simulink model "seven_level_NPC_MLI_Inverter"  (R2022a)
settings: Solver=VariableStepAuto  StartTime=0.0  StopTime=0.02  RelTol=1e-3
libraries: spsDiodeLib x30, spsVoltageMeasurementLib x13, spsIGBTDiodeLib x12, spsDCVoltageSourceLib x6, simulink x6, spsCurrentMeasurementLib x1, spsSeriesRLCBranchLib x1, spspowerguiLib x1
settings Model: Creator=P.O.M.G  LastModifiedBy=P.O.M.G

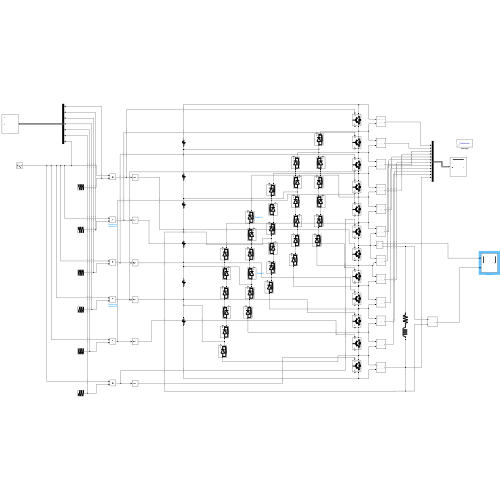
[thumbnail: Simulink's stored preview of the top-level diagram]
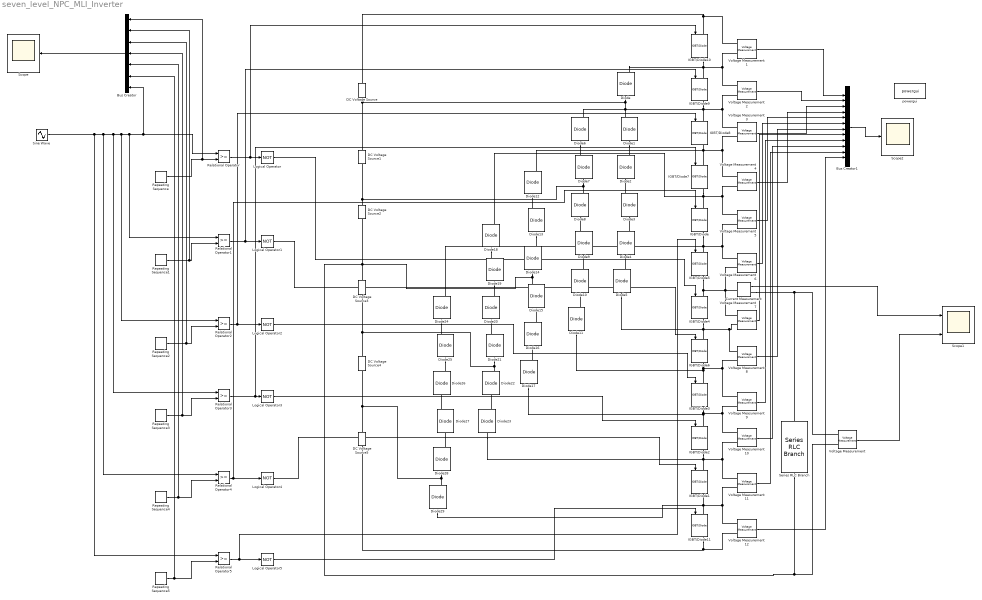
== system seven_level_NPC_MLI_Inverter ==
  Bus Creator : BusCreator  Inputs=7
  Bus Creator1 : BusCreator  Inputs=12
  Current Measurement : spsCurrentMeasurementLib/Current Measurement  PhasorSimulation=off  OutputType=Complex  PSBequivalent=0
  DC Voltage Source{,1..5} (6 alike) : spsDCVoltageSourceLib/DC Voltage Source  Amplitude=100  Measurements=None
  Diode{,1..29} (30 alike) : spsDiodeLib/Diode  Ron=0.001  Lon=0  Vf=0.8  IC=0  UseSnubber=0  Rs=500  Cs=250e-9  Measurements=on
  IGBT/Diode{,1..11} (12 alike) : spsIGBTDiodeLib/IGBT//Diode  Ron=1e-3  Rs=1e5  Cs=inf  Measurements=on
  Logical Operator{,1..5} (6 alike) : Logic  Operator=NOT  AllPortsSameDT=off  OutDataTypeStr=boolean
  Relational Operator{,1..5} (6 alike) : RelationalOperator  OutDataTypeStr=boolean  RndMeth=Simplest  InputSameDT=off
  Repeating Sequence : simulink/Sources/Repeating Sequence  rep_seq_t=[0 0.5 1]/500  rep_seq_y=[1, 0, -1]
  Repeating Sequence1 : simulink/Sources/Repeating Sequence  rep_seq_t=[0 0.5 1]/500  rep_seq_y=[0, 1, -1]
  Repeating Sequence2 : simulink/Sources/Repeating Sequence  rep_seq_t=[0 0.5 1]/500  rep_seq_y=[-1, 1, 0]
  Repeating Sequence3 : simulink/Sources/Repeating Sequence  rep_seq_t=[0 0.5 1]/500  rep_seq_y=[-1, 0, 1]
  Repeating Sequence4 : simulink/Sources/Repeating Sequence  rep_seq_t=[0 0.5 1]/500  rep_seq_y=[1, -1, 0]
  Repeating Sequence5 : simulink/Sources/Repeating Sequence  rep_seq_t=[0 0.5 1]/500  rep_seq_y=[0, -1, 1]
  Scope : Scope
  Scope1 : Scope  NumInputPorts=2
  Scope2 : Scope
  Series RLC Branch : spsSeriesRLCBranchLib/Series RLC Branch  LConnTagsString=__new0  RConnTagsString=__new0  BranchType=RL  Resistance=5  Inductance=5e-3  SetiL0=off  InitialCurrent=0  Capacitance=1e-6  Setx0=off  InitialVoltage=0  Measurements=None
  Sine Wave : Sin  Amplitude=0.9  Frequency=2*pi*50  SampleTime=0
  Voltage Measurement{,1..12} (13 alike) : spsVoltageMeasurementLib/Voltage Measurement  PhasorSimulation=off  OutputType=Complex  PSBequivalent=0
  powergui : spspowerguiLib/powergui  Priority=1  SimulationMode=Continuous  SampleTime=50e-6  frequency=60  Iterations=50  frequencyindice=0  Pbase=100e6  ErrMax=1e-4  UnitsV=kV  UnitsW=MW  buscounter=0  FunctionMessages=off  echomessages=off  EnableUseOfTLC=off  CurrentSourceSwitches=off  DisableSnubberDevices=off  DisableRonSwitches=off  DisableVfSwitches=off  DisplayEquations=off  AutomaticDiscreteSolvers=off  SolverType=Tustin/Backward Euler (TBE)  Interpol=off  ExternalGateDelay=off  methode=off  Ts=100  x0status=blocks  SPID=on  SwTol=0  HookPort=off  NonlinearTolerance=1e-4  nMaxIteration=100  ContinueOnMaxIteration=off  RestoreLinks=warning  ResistiveCurrentMeasurement=off  Frange=[0:2:500]  Ylog=off  Xlog=on  ShowGrid=off  save=off  variable=ZData  structure=0  ZoomFFT=off  StartTime=0.0  cycles=1  DisplayStyle=1  fundamental=60  FreqAxis=off  MaxFrequency=1000  frequencyindicesteady=1  RmsSteady=1  display=off
  wires:
  Repeating Sequence/1 -> Relational Operator/2, Bus Creator/1
  Relational Operator/1 -> IGBT/Diode10/1, Logical Operator/1
  Repeating Sequence1/1 -> Relational Operator1/2, Bus Creator/2
  Relational Operator1/1 -> IGBT/Diode9/1, Logical Operator1/1
  Repeating Sequence2/1 -> Bus Creator/3, Relational Operator2/2
  Relational Operator3/1 -> IGBT/Diode7/1, Logical Operator3/1
  Repeating Sequence3/1 -> Bus Creator/4, Relational Operator3/2
  Relational Operator4/1 -> Logical Operator4/1, IGBT/Diode/1
  Repeating Sequence4/1 -> Bus Creator/5, Relational Operator4/2
  Repeating Sequence5/1 -> Bus Creator/6, Relational Operator5/2
  Relational Operator5/1 -> IGBT/Diode5/1, Logical Operator5/1
  Sine Wave/1 -> Relational Operator5/1, Relational Operator4/1, Relational Operator3/1, Relational Operator2/1, Relational Operator1/1, Bus Creator/7, Relational Operator/1
  Relational Operator2/1 -> Logical Operator2/1, IGBT/Diode8/1
  Logical Operator/1 -> IGBT/Diode4/1
  Logical Operator1/1 -> IGBT/Diode6/1
  Logical Operator2/1 -> IGBT/Diode3/1
  Logical Operator3/1 -> IGBT/Diode2/1
  Logical Operator4/1 -> IGBT/Diode1/1
  Logical Operator5/1 -> IGBT/Diode11/1
  Bus Creator/1 -> Scope/1
  Current Measurement/1 -> Scope1/1
  Voltage Measurement/1 -> Scope1/2
  Bus Creator1/1 -> Scope2/1
  Voltage Measurement1/1 -> Bus Creator1/1
  Voltage Measurement2/1 -> Bus Creator1/2
  Voltage Measurement3/1 -> Bus Creator1/3
  Voltage Measurement4/1 -> Bus Creator1/4
  Voltage Measurement5/1 -> Bus Creator1/5
  Voltage Measurement6/1 -> Bus Creator1/6
  Voltage Measurement7/1 -> Bus Creator1/8
  Voltage Measurement8/1 -> Bus Creator1/7
  Voltage Measurement9/1 -> Bus Creator1/9
  Voltage Measurement10/1 -> Bus Creator1/10
  Voltage Measurement11/1 -> Bus Creator1/11
  Voltage Measurement12/1 -> Bus Creator1/12
  connections:
  IGBT/Diode8/RConn1 -- Voltage Measurement3/LConn2 -- Voltage Measurement4/LConn1 -- Diode12/RConn1 -- IGBT/Diode7/LConn1
  IGBT/Diode9/RConn1 -- Voltage Measurement2/LConn2 -- Voltage Measurement3/LConn1 -- Diode/LConn1 -- DC Voltage Source1/RConn1 -- DC Voltage Source/LConn1 -- Diode1/RConn1 -- Diode6/RConn1 -- IGBT/Diode8/LConn1
  IGBT/Diode10/RConn1 -- Voltage Measurement2/LConn1 -- Voltage Measurement1/LConn2 -- Diode/RConn1 -- IGBT/Diode9/LConn1
  IGBT/Diode11/LConn1 -- Voltage Measurement12/LConn1 -- Voltage Measurement11/LConn2 -- Diode29/LConn1 -- IGBT/Diode1/RConn1
  DC Voltage Source2/RConn1 -- Diode8/RConn1 -- Diode7/LConn1 -- DC Voltage Source1/LConn1
  DC Voltage Source3/RConn1 -- Voltage Measurement/LConn2 -- Series RLC Branch/RConn1 -- Diode15/RConn1 -- Diode14/LConn1 -- DC Voltage Source2/LConn1
  DC Voltage Source4/RConn1 -- Diode21/LConn1 -- Diode22/RConn1 -- DC Voltage Source3/LConn1
  DC Voltage Source5/RConn1 -- Diode28/LConn1 -- Diode29/RConn1 -- DC Voltage Source4/LConn1
  DC Voltage Source/RConn1 -- Voltage Measurement1/LConn1 -- IGBT/Diode10/LConn1
  IGBT/Diode11/RConn1 -- Voltage Measurement12/LConn2 -- DC Voltage Source5/LConn1
  IGBT/Diode7/RConn1 -- Voltage Measurement5/LConn1 -- Voltage Measurement4/LConn2 -- IGBT/Diode/LConn1 -- Diode18/RConn1
  IGBT/Diode/RConn1 -- Voltage Measurement5/LConn2 -- Voltage Measurement6/LConn1 -- Diode24/RConn1 -- IGBT/Diode5/LConn1
  IGBT/Diode5/RConn1 -- Voltage Measurement7/LConn1 -- Voltage Measurement6/LConn2 -- Current Measurement/LConn1 -- IGBT/Diode4/LConn1
  IGBT/Diode4/RConn1 -- Voltage Measurement8/LConn1 -- Voltage Measurement7/LConn2 -- Diode5/LConn1 -- IGBT/Diode6/LConn1
  IGBT/Diode6/RConn1 -- Voltage Measurement8/LConn2 -- Voltage Measurement9/LConn1 -- Diode11/LConn1 -- IGBT/Diode3/LConn1
  IGBT/Diode3/RConn1 -- Voltage Measurement9/LConn2 -- Voltage Measurement10/LConn1 -- Diode17/LConn1 -- IGBT/Diode2/LConn1
  IGBT/Diode2/RConn1 -- Voltage Measurement10/LConn2 -- Voltage Measurement11/LConn1 -- Diode23/LConn1 -- IGBT/Diode1/LConn1
  Diode1/LConn1 -- Diode2/RConn1
  Diode3/RConn1 -- Diode2/LConn1
  Diode4/RConn1 -- Diode3/LConn1
  Diode5/RConn1 -- Diode4/LConn1
  Diode6/LConn1 -- Diode7/RConn1
  Diode9/RConn1 -- Diode8/LConn1
  Diode10/RConn1 -- Diode9/LConn1
  Diode11/RConn1 -- Diode10/LConn1
  Diode12/LConn1 -- Diode13/RConn1
  Diode13/LConn1 -- Diode14/RConn1
  Diode16/RConn1 -- Diode15/LConn1
  Diode17/RConn1 -- Diode16/LConn1
  Diode18/LConn1 -- Diode19/RConn1
  Diode21/RConn1 -- Diode20/LConn1
  Diode19/LConn1 -- Diode20/RConn1
  Diode23/RConn1 -- Diode22/LConn1
  Diode24/LConn1 -- Diode25/RConn1
  Diode27/RConn1 -- Diode26/LConn1
  Diode25/LConn1 -- Diode26/RConn1
  Diode28/RConn1 -- Diode27/LConn1
  Current Measurement/RConn1 -- Voltage Measurement/LConn1 -- Series RLC Branch/LConn1
